simulink model "wjcgzq"  (Simulink 6.0)
settings: Solver=ode45  StartTime=0.0  StopTime=7  MaxStep=0.003  RelTol=1e-3
InitFcn:
  | tracker()
values from neighbouring files (symbols this model uses):
  A = [           0                   1 0             0;     (M+m)*m*g*l/((M+m)*I+M*m*l^2) 0 0 m*l*b/((M+m)*I+M*m*l^2);               0                   0 0             1;      -m^2*l^2*g/((M+m)*I+M*m*l^2) 0 0 -(I+m*l^2)*b/((M+m)*I+M*m*l^2)]    [pendulum.m]    (also in tracker.m = [0 1 0 0;51.58 0 0 0.5263;0 0 0 1;-7.737 0 0 -0.1789])
  B = [0;-m*l/(((M+m)*I+M*m*l^2));0;(I+m*l^2)/((M+m)*I+M*m*l^2)]    [pendulum.m]    (also in tracker.m = [0;-5.263;0;1.789])
  C = [0 0 1 0;1 0 0 0]    [pendulum.m]    (also in tracker.m = [0 0 1 0])
  K = place(A22',A12',Pole)    [jwgcl.m]    (also in jwgcp.m; tracker.m = Kt(:,1:4))
  Kc = -Kt(:,5)    [tracker.m]
settings Model: LastModifiedBy=Administrator

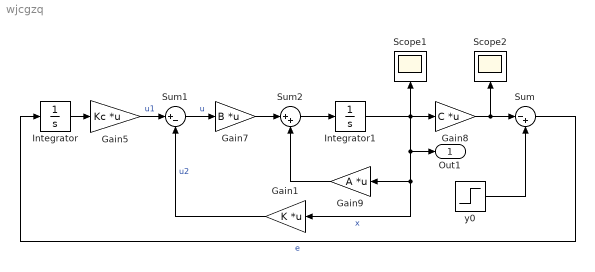
== system wjcgzq ==
  Gain1 : Gain  Orientation=left  Gain=K  Multiplication=Matrix(K*u)  SaturateOnIntegerOverflow=on
  Gain5 : Gain  Gain=Kc  Multiplication=Matrix(K*u)
  Gain7 : Gain  Gain=B  Multiplication=Matrix(K*u)  SaturateOnIntegerOverflow=on
  Gain8 : Gain  Gain=C  Multiplication=Matrix(K*u)  SaturateOnIntegerOverflow=on
  Gain9 : Gain  Orientation=left  Gain=A  Multiplication=Matrix(K*u)  SaturateOnIntegerOverflow=on
  Integrator : Integrator
  Integrator1 : Integrator
  Scope1 : Scope
      settings: Orientation=up
  Scope2 : Scope
      settings: Orientation=up
  Sum : Sum  Inputs=|-+
  Sum1 : Sum  Inputs=|+-
  Sum2 : Sum  Inputs=|++
  y0 : Step  Time=0  After=0.2  SampleTime=0
  Out1 : Outport
  wires:
  Sum/1 -> Integrator/1  "e"
  Gain5/1 -> Sum1/1  "u1"
  Gain7/1 -> Sum2/1
  Sum2/1 -> Integrator1/1
  Integrator1/1 -> Gain8/1, Scope1/1, Gain9/1, Gain1/1, Out1/1  "x"
  Gain9/1 -> Sum2/2
  Sum1/1 -> Gain7/1  "u"
  Gain1/1 -> Sum1/2  "u2"
  Gain8/1 -> Scope2/1, Sum/1
  Integrator/1 -> Gain5/1
  y0/1 -> Sum/2
